simulink model "Wm"  (R2016a)
settings: Solver=VariableStepAuto  StartTime=0.0  StopTime=10.0  RelTol=1e-3
undefined symbols (not defined in the file): Tem, Tloss
settings Model: Creator=hi  LastModifiedBy=hi

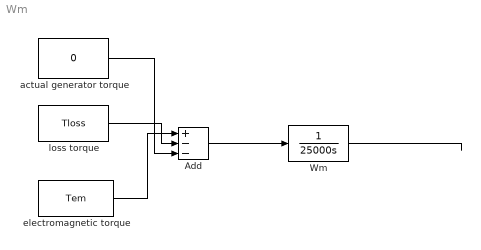
== system Wm ==
  " actual generator torque " : Constant  Value=0
  Add : Sum  Inputs=+--
  Wm : TransferFcn  Denominator=[25000 0]
  electromagnetic torque : Constant  Value=Tem
  "loss torque " : Constant  Value=Tloss
  wires:
  electromagnetic torque/1 -> Add/1
  "loss torque "/1 -> Add/2
  " actual generator torque "/1 -> Add/3
  Add/1 -> Wm/1
  Wm/1 -> ?
